simulink model "BUCK_CHOPPER_OL"  (R2024a)
settings: Solver=VariableStepAuto  StartTime=0.0  StopTime=0.2  RelTol=1e-3
libraries: spsCurrentMeasurementLib x3, spsMeanLib x3, spsVoltageMeasurementLib x3, spsDCVoltageSourceLib x2, spsSeriesRLCBranchLib x2, spsDCMachineLib x1, spsDiodeLib x1, spsMosfetLib x1, sps_lib x1
settings Model: Creator=sreet  LastModifiedBy=sreet

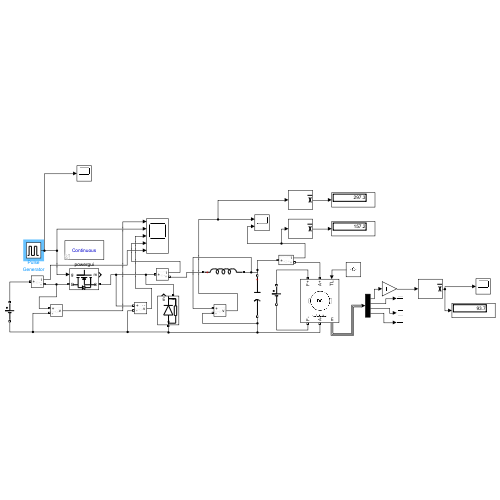
[thumbnail: Simulink's stored preview of the top-level diagram]
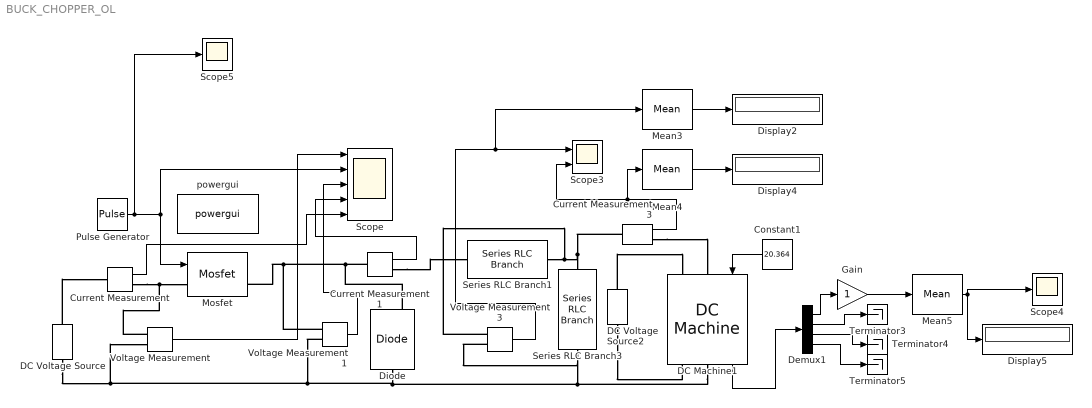
== system BUCK_CHOPPER_OL ==
  Constant1 : Constant  Value=20.364
  Current Measurement : spsCurrentMeasurementLib/Current Measurement  PhasorSimulation=off  OutputType=Complex  PSBequivalent=0
  Current Measurement1 : spsCurrentMeasurementLib/Current Measurement  PhasorSimulation=off  OutputType=Complex  PSBequivalent=0
  Current Measurement3 : spsCurrentMeasurementLib/Current Measurement  PhasorSimulation=off  OutputType=Complex  PSBequivalent=0
  DC Machine1 : spsDCMachineLib/DC Machine  PresetModel=No  MechanicalLoad=Torque TL  FieldType=Wound  ShowDetailedParameters=on  MeasurementBus=off  RLa="[ 0.6  0.012]"  RLf="[ 240  120]"  Laf=1.8  MachineConstant=Torque constant (N.m/A)  Ke=1.8  Kt=1.8  J=1  Bm=0  Tf=0  w0=1  Ifinit=1.25  TsPowergui=0  TsBlock=-1
  DC Voltage Source : spsDCVoltageSourceLib/DC Voltage Source  Amplitude=380  Measurements=None
  DC Voltage Source2 : spsDCVoltageSourceLib/DC Voltage Source  Amplitude=300  Measurements=None
  Demux1 : Demux
  Diode : spsDiodeLib/Diode  Ron=0.001  Lon=0  Vf=0.8  IC=0  UseSnubber=0  Rs=500  Cs=250e-9  Measurements=on
  Display2 : Display
  Display4 : Display
  Display5 : Display
  Gain : Gain
  Mean3 : spsMeanLib/Mean  Freq=60  Vinit=0  Ts=0
  Mean4 : spsMeanLib/Mean  Freq=60  Vinit=0  Ts=0
  Mean5 : spsMeanLib/Mean  Freq=60  Vinit=0  Ts=0
  Mosfet : spsMosfetLib/Mosfet  Ron=0.1  Lon=0  Rd=0.01  Vfd=0  IC=0  Rs=1e5  Cs=inf  Measurements=on
  Pulse Generator : DiscretePulseGenerator  PulseType=Time based  Amplitude=10  Period=0.02  PulseWidth=50
  Scope : Scope  NumInputPorts=5
  Scope3 : Scope  NumInputPorts=2
  Scope4 : Scope
  Scope5 : Scope
  Series RLC Branch1 : spsSeriesRLCBranchLib/Series RLC Branch  LConnTagsString=__new0  RConnTagsString=__new0  BranchType=L  Resistance=1  Inductance=1e-3  SetiL0=off  InitialCurrent=0  Capacitance=1e-6  Setx0=off  InitialVoltage=0  Measurements=None
  Series RLC Branch3 : spsSeriesRLCBranchLib/Series RLC Branch  LConnTagsString=__new0  RConnTagsString=__new0  BranchType=C  Resistance=1  Inductance=1e-3  SetiL0=off  InitialCurrent=0  Capacitance=100e-3  Setx0=off  InitialVoltage=0  Measurements=None
  Terminator3 : Terminator
  Terminator4 : Terminator
  Terminator5 : Terminator
  Voltage Measurement : spsVoltageMeasurementLib/Voltage Measurement  PhasorSimulation=off  OutputType=Complex  PSBequivalent=0
  Voltage Measurement1 : spsVoltageMeasurementLib/Voltage Measurement  PhasorSimulation=off  OutputType=Complex  PSBequivalent=0
  Voltage Measurement3 : spsVoltageMeasurementLib/Voltage Measurement  PhasorSimulation=off  OutputType=Complex  PSBequivalent=0
  powergui : sps_lib/powergui  Priority=1  SimulationMode=Continuous  SampleTime=50e-6  frequency=60  Iterations=50  frequencyindice=0  Pbase=100e6  ErrMax=1e-4  UnitsV=kV  UnitsW=MW  buscounter=0  FunctionMessages=off  echomessages=off  EnableUseOfTLC=off  CurrentSourceSwitches=off  DisableSnubberDevices=off  DisableRonSwitches=off  DisableVfSwitches=off  DisplayEquations=off  AutomaticDiscreteSolvers=off  SolverType=Tustin/Backward Euler (TBE)  Interpol=off  ExternalGateDelay=off  methode=off  Ts=100  x0status=blocks  SPID=on  SwTol=0  HookPort=off  NonlinearTolerance=1e-4  nMaxIteration=100  ContinueOnMaxIteration=off  RestoreLinks=warning  ResistiveCurrentMeasurement=off  Frange=[0:2:500]  Ylog=off  Xlog=on  ShowGrid=off  save=off  variable=ZData  structure=0  ZoomFFT=off  StartTime=0.0  cycles=1  DisplayStyle=1  fundamental=60  FreqAxis=off  MaxFrequency=1000  frequencyindicesteady=1  RmsSteady=1  display=off
  wires:
  Pulse Generator/1 -> Scope5/1, Scope/2, Mosfet/1
  Voltage Measurement/1 -> Scope/1
  Voltage Measurement1/1 -> Scope/3
  Current Measurement1/1 -> Scope/4
  Voltage Measurement3/1 -> Mean3/1, Scope3/1
  Current Measurement3/1 -> Mean4/1, Scope3/2
  Mean4/1 -> Display4/1
  Mean3/1 -> Display2/1
  Constant1/1 -> DC Machine1/1
  DC Machine1/1 -> Demux1/1
  Demux1/1 -> Gain/1
  Demux1/2 -> Terminator3/1
  Demux1/3 -> Terminator4/1
  Demux1/4 -> Terminator5/1
  Gain/1 -> Mean5/1
  Mean5/1 -> Display5/1, Scope4/1
  Current Measurement/1 -> Scope/5
  connections:
  DC Voltage Source/RConn1 -- Current Measurement/LConn1
  Current Measurement/RConn1 -- Voltage Measurement/LConn1 -- Mosfet/LConn1
  DC Voltage Source/LConn1 -- Voltage Measurement3/LConn2 -- Series RLC Branch3/RConn1 -- DC Machine1/RConn1 -- Diode/LConn1 -- Voltage Measurement1/LConn2 -- Voltage Measurement/LConn2
  Current Measurement1/LConn1 -- Voltage Measurement1/LConn1 -- Mosfet/RConn1 -- Diode/RConn1
  Series RLC Branch1/RConn1 -- Voltage Measurement3/LConn1 -- Current Measurement3/LConn1 -- Series RLC Branch3/LConn1
  Current Measurement1/RConn1 -- Series RLC Branch1/LConn1
  DC Voltage Source2/RConn1 -- DC Machine1/LConn2
  DC Voltage Source2/LConn1 -- DC Machine1/RConn2
  Current Measurement3/RConn1 -- DC Machine1/LConn1
